simulink model "quadrotorsmodel2"  (R2025b)
settings: Solver=FixedStepAuto  StartTime=0.0  StopTime=SimulationTime  FixedStep=timestep  RelTol=1e-3
values from neighbouring files (symbols this model uses):
  alt_init = 0    [data_hard.mat]
  fense_lats = [14.294404 14.301206]    [data_hard.mat]
  fense_lons = [101.16723 101.176794]    [data_hard.mat]
  g = 9.81    [Copy_of_TESA_Workspace2.m]    (also in TESA_Workspace2.m)
  I = eye(3,3)    [Copy_of_TESA_Workspace2.m]    (also in TESA_Workspace2.m)
  K = [ 1   1   1   1 ... (first row only)    [Copy_of_TESA_Workspace2.m]    (also in TESA_Workspace2.m)
  lat_init = 14.303    [data_hard.mat]
  long_init = 101.155    [data_hard.mat]
  m = 4.34    [Copy_of_TESA_Workspace2.m]    (also in TESA_Workspace2.m)
undefined symbols (not defined in the file or in its folder): dspblkCoreblockFVToolHelper, fractalcoef, gcbh, Kp, Kr, Kv, Kw
libraries: sensorgpslib x1, mspsensorlib x1
settings Model: Creator=worap  LastModifiedBy=Gigabyte
settings DataIOCC: ExternalInput=inputStructure  LoadExternalInput=on

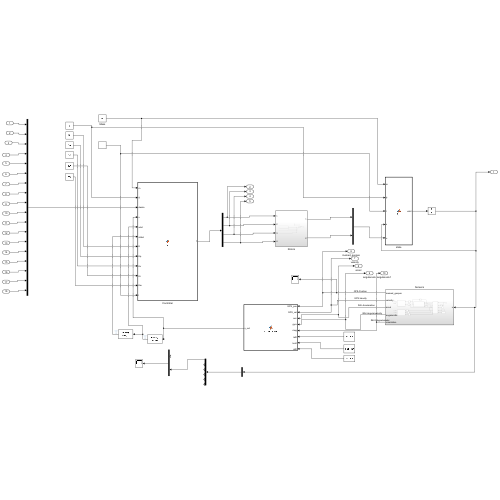
[thumbnail: Simulink's stored preview of the top-level diagram]
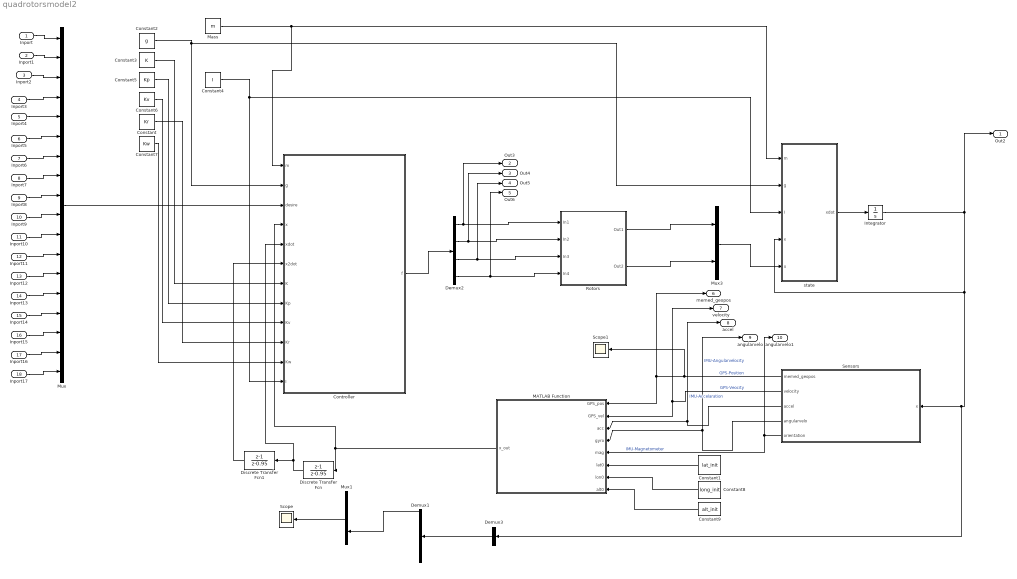
== system quadrotorsmodel2 ==
  Inport : Inport
  Inport1 : Inport  Port=2
  Inport2 : Inport  Port=3
  Inport3 : Inport  Port=4
  Inport4 : Inport  Port=5
  Inport5 : Inport  Port=6
  Inport6 : Inport  Port=7
  Inport7 : Inport  Port=8
  Inport8 : Inport  Port=9
  Inport9 : Inport  Port=10
  Inport10 : Inport  Port=11
  Inport11 : Inport  Port=12
  Inport12 : Inport  Port=13
  Inport13 : Inport  Port=14
  Inport14 : Inport  Port=15
  Inport15 : Inport  Port=16
  Inport16 : Inport  Port=17
  Inport17 : Inport  Port=18
  Constant : Constant  Value=Kr
  Constant1 : Constant  Value=lat_init
  Constant2 : Constant  Value=g
  Constant3 : Constant  Value=K
  Constant4 : Constant  Value=I
  Constant5 : Constant  Value=Kp
  Constant6 : Constant  Value=Kv
  Constant7 : Constant  Value=Kw
  Constant8 : Constant  Value=long_init
  Constant9 : Constant  Value=alt_init
  Controller : MATLAB Function  TreatAsAtomicUnit=on
  Demux1 : Demux  Outputs=6
  Demux2 : Demux
  Demux3 : Demux  Outputs=1
  Discrete Transfer Fcn : DiscreteTransferFcn  LoadFcn=dspblkCoreblockFVToolHelper(gcbh,'load');  Numerator="[1  -1]"  Denominator="[1  -0.95]"  InitialStates=0.01
      settings: CopyFcn=dspblkCoreblockFVToolHelper(gcbh,'copy');  DeleteFcn=dspblkCoreblockFVToolHelper(gcbh,'close');  ModelCloseFcn=dspblkCoreblockFVToolHelper(gcbh,'close');  PreSaveFcn=dspblkCoreblockFVToolHelper(gcbh,'presave');  PostSaveFcn=dspblkCoreblockFVToolHelper(gcbh,'postsave');  CloseFcn=dspblkCoreblockFVToolHelper(gcbh,'close');
  Discrete Transfer Fcn1 : DiscreteTransferFcn  LoadFcn=dspblkCoreblockFVToolHelper(gcbh,'load');  Numerator="[1  -1]"  Denominator="[1  -0.95]"  InitialStates=0.01
      settings: CopyFcn=dspblkCoreblockFVToolHelper(gcbh,'copy');  DeleteFcn=dspblkCoreblockFVToolHelper(gcbh,'close');  ModelCloseFcn=dspblkCoreblockFVToolHelper(gcbh,'close');  PreSaveFcn=dspblkCoreblockFVToolHelper(gcbh,'presave');  PostSaveFcn=dspblkCoreblockFVToolHelper(gcbh,'postsave');  CloseFcn=dspblkCoreblockFVToolHelper(gcbh,'close');
  Integrator : Integrator  InitialCondition=[0;0;0;0;0;0;1;0;0;0;1;0;0;0;1;0;0;0]
  MATLAB Function : MATLAB Function  TreatAsAtomicUnit=on
  Mass : Constant  Value=m
  Mux : Mux  Inputs=18
  Mux1 : Mux  Inputs=2
  Mux3 : Mux  Inputs=2
  Rotors : Subsystem
  Scope : Scope
      settings: ActiveDisplayYMinimum=-1789.9407  ActiveDisplayYMaximum=2269.5419
  Scope1 : Scope
      settings: ActiveDisplayYMinimum=-1789.9407  ActiveDisplayYMaximum=2269.5419
  Sensors : Subsystem
  state : MATLAB Function  TreatAsAtomicUnit=on
  Out2 : Outport
  Out3 : Outport  Port=2
  Out4 : Outport  Port=3
  Out5 : Outport  Port=4
  Out6 : Outport  Port=5
  memed_geopos : Outport  Port=6
  velocity : Outport  Port=7
  accel : Outport  Port=8
  angularvelo : Outport  Port=9
  angularvelo1 : Outport  Port=10
  wires:
  Mass/1 -> state/1(m), Controller/1(m)
  Demux2/2 -> Out4/1, Rotors/2(In2)
  Rotors/1(Out1) -> Mux3/1
  Rotors/2(Out2) -> Mux3/2
  Demux2/3 -> Out5/1, Rotors/3(In3)
  Demux2/4 -> Out6/1, Rotors/4(In4)
  Constant4/1 -> state/3(I), Controller/12(I)
  Controller/1(f) -> Demux2/1
  Demux2/1 -> Out3/1, Rotors/1(In1)
  Constant2/1 -> state/2(g), Controller/2(g)
  Constant3/1 -> Controller/7(K)
  Constant5/1 -> Controller/8(Kp)
  Constant6/1 -> Controller/9(Kv)
  Constant7/1 -> Controller/11(Kw)
  Constant/1 -> Controller/10(Kr)
  Mux3/1 -> state/5(u)
  state/1(xdot) -> Integrator/1
  Mux/1 -> Controller/3(desire)
  Inport17/1 -> Mux/18
  Inport16/1 -> Mux/17
  Inport15/1 -> Mux/16
  Inport14/1 -> Mux/15
  Inport13/1 -> Mux/14
  Inport12/1 -> Mux/13
  Inport11/1 -> Mux/12
  Inport10/1 -> Mux/11
  Inport9/1 -> Mux/10
  Inport8/1 -> Mux/9
  Inport7/1 -> Mux/8
  Inport6/1 -> Mux/7
  Inport5/1 -> Mux/6
  Inport4/1 -> Mux/5
  Inport3/1 -> Mux/4
  Inport2/1 -> Mux/3
  Inport1/1 -> Mux/2
  Inport/1 -> Mux/1
  Sensors/1(memed_geopos) -> Scope1/1, MATLAB Function/1(GPS_pos), memed_geopos/1  "GPS-Position"
  Sensors/2(velocity) -> MATLAB Function/2(GPS_vel), velocity/1  "GPS-Veocity"
  Sensors/3(accel) -> MATLAB Function/3(acc), accel/1  "IMU-Accelaration"
  Sensors/4(angularvelo) -> angularvelo/1, MATLAB Function/4(gyro)  "IMU-Angularvelocity"
  Sensors/5(orientation) -> MATLAB Function/5(mag), angularvelo1/1  "IMU-Magnetometer"
  Discrete Transfer Fcn1/1 -> Controller/6(x2dot)
  Integrator/1 -> Demux3/1, Sensors/1(x), state/4(x), Out2/1
  Mux1/1 -> Scope/1
  MATLAB Function/1(x_out) -> Controller/4(x), Discrete Transfer Fcn/1
  Constant1/1 -> MATLAB Function/6(lat0)
  Constant8/1 -> MATLAB Function/7(lon0)
  Constant9/1 -> MATLAB Function/8(alt0)
  Demux1/1 -> Mux1/2
  Demux3/1 -> Demux1/1
  Discrete Transfer Fcn/1 -> Controller/5(xdot), Discrete Transfer Fcn1/1

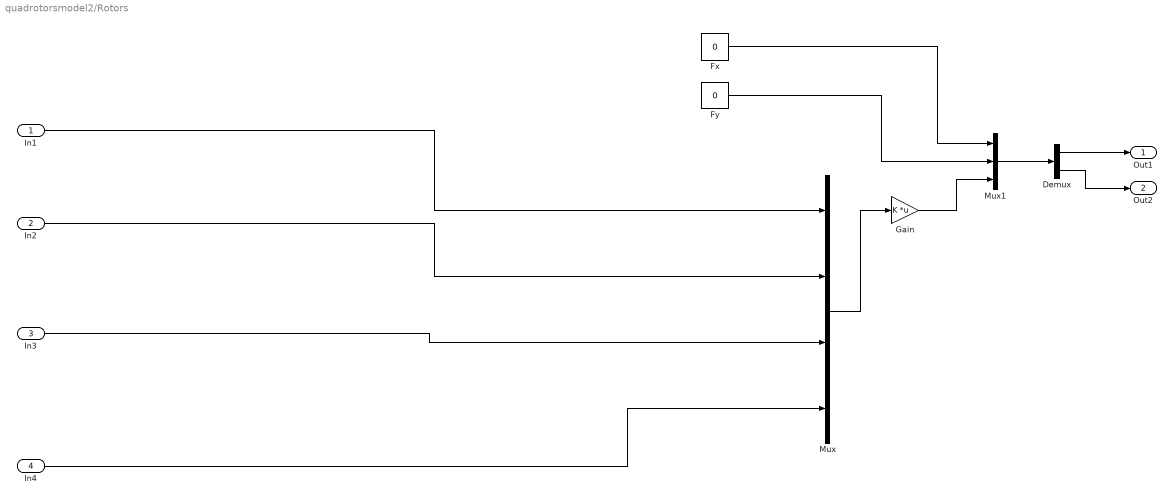
== system quadrotorsmodel2/Rotors ==
  In1 : Inport
  In2 : Inport  Port=2
  In3 : Inport  Port=3
  In4 : Inport  Port=4
  Demux : Demux  Outputs=2
  Fx : Constant  Value=0
  Fy : Constant  Value=0
  Gain : Gain  Gain=K  Multiplication=Matrix(K*u) (u vector)
  Mux : Mux
  Mux1 : Mux  Inputs=3
  Out1 : Outport
  Out2 : Outport  Port=2
  wires:
  Fx/1 -> Mux1/1
  Mux1/1 -> Demux/1
  Fy/1 -> Mux1/2
  Mux/1 -> Gain/1
  Gain/1 -> Mux1/3
  Demux/2 -> Out2/1
  Demux/1 -> Out1/1
  In1/1 -> Mux/1
  In2/1 -> Mux/2
  In3/1 -> Mux/3
  In4/1 -> Mux/4

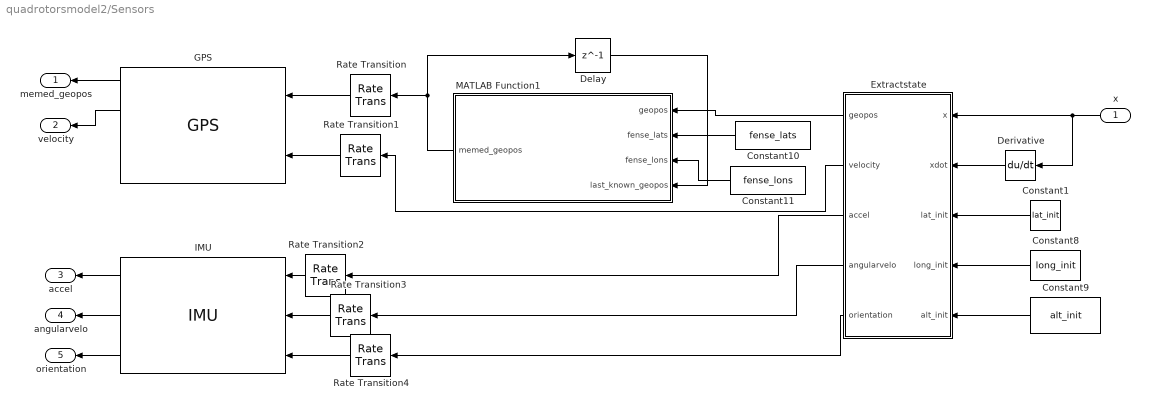
== system quadrotorsmodel2/Sensors ==
  x : Inport
  Constant1 : Constant  Value=lat_init
  Constant10 : Constant  Value=fense_lats
  Constant11 : Constant  Value=fense_lons
  Constant8 : Constant  Value=long_init
  Constant9 : Constant  Value=alt_init
  Delay : Delay  DelayLength=1  InitialCondition=0
  Derivative : Derivative
  Extractstate : MATLAB Function  TreatAsAtomicUnit=on
  GPS : sensorgpslib/GPS  DispRefFrame=NED  PositionInputFormat=Geodetic  ReferenceLocation=[ 0, 0, 0 ]  HorizontalPositionAccuracy=1.6  VerticalPositionAccuracy=3  VelocityAccuracy=0.1  DecayFactor=0.999  SeedDouble=67  SimulateUsing=Interpreted execution
      settings: LibrarySourceBlock=mspsensorlib/GPS
  IMU : mspsensorlib/IMU  DispRefFrame=NED  TemperaturePort=off  Temperature=25  MagneticFieldPort=off  MagneticFieldNED=[ 27.5550, -2.4169, -16.0849 ]  MagneticFieldENU=[ -2.4169, 27.5550, 16.0849 ]  SeedDouble=67  SimulateUsing=Interpreted execution  AccelParamsMeasurementRange=Inf  AccelParamsResolution=0  AccelParamsConstantBias=[ 0, 0, 0 ]  AccelParamsAxesMisalignment=[ 100, 0, 0; 0, 100, 0; 0, 0, 100 ]  AccelParamsNoiseDensity=[ 0.003924 0.003924 0.003924 ]  AccelParamsBiasInstability=[ 0, 0, 0 ]  AccelParamsBiasInstabilityNumerator=fractalcoef().Numerator  AccelParamsBiasInstabilityDenominator=fractalcoef().Denominator  AccelParamsRandomWalk=[ 0, 0, 0 ]  AccelParamsNoiseType=double-sided  AccelParamsTemperatureBias=[ 0, 0, 0 ]  AccelParamsTemperatureScaleFactor=[ 0, 0, 0 ]  GyroParamsMeasurementRange=Inf  GyroParamsResolution=0  GyroParamsConstantBias=[ 0, 0, 0 ]  GyroParamsAxesMisalignment=[ 100, 0, 0; 0, 100, 0; 0, 0, 100 ]  GyroParamsAccelerationBias=[ 0, 0, 0 ]  GyroParamsNoiseDensity=[ 0.0125, 0.0125, 0.0125 ]  GyroParamsBiasInstability=[ 0, 0, 0 ]  GyroParamsBiasInstabilityNumerator=fractalcoef().Numerator  GyroParamsBiasInstabilityDenominator=fractalcoef().Denominator  GyroParamsRandomWalk=[ 0, 0, 0 ]  GyroParamsNoiseType=double-sided  GyroParamsTemperatureBias=[ 0, 0, 0 ]  GyroParamsTemperatureScaleFactor=[ 0, 0, 0 ]  MagParamsMeasurementRange=Inf  MagParamsResolution=0  MagParamsConstantBias=[ 0, 0, 0 ]  MagParamsAxesMisalignment=[ 100, 0, 0; 0, 100, 0; 0, 0, 100 ]  MagParamsNoiseDensity=[0.6 0.6 0.9]/sqrt(100)  MagParamsBiasInstability=[ 0, 0, 0 ]  MagParamsBiasInstabilityNumerator=fractalcoef().Numerator  MagParamsBiasInstabilityDenominator=fractalcoef().Denominator  MagParamsRandomWalk=[ 0, 0, 0 ]  MagParamsNoiseType=double-sided  MagParamsTemperatureBias=[ 0, 0, 0 ]  MagParamsTemperatureScaleFactor=[ 0, 0, 0 ]
  MATLAB Function1 : MATLAB Function  TreatAsAtomicUnit=on
  Rate Transition{,1..4} (5 alike) : RateTransition
  memed_geopos : Outport
  velocity : Outport  Port=2
  accel : Outport  Port=3
  angularvelo : Outport  Port=4
  orientation : Outport  Port=5
  wires:
  Constant11/1 -> MATLAB Function1/3(fense_lons)
  Constant8/1 -> Extractstate/4(long_init)
  Constant1/1 -> Extractstate/3(lat_init)
  Constant10/1 -> MATLAB Function1/2(fense_lats)
  Delay/1 -> MATLAB Function1/4(last_known_geopos)
  Derivative/1 -> Extractstate/2(xdot)
  Constant9/1 -> Extractstate/5(alt_init)
  MATLAB Function1/1(memed_geopos) -> Rate Transition/1, Delay/1
  x/1 -> Derivative/1, Extractstate/1(x)
  IMU/1 -> accel/1
  IMU/2 -> angularvelo/1
  IMU/3 -> orientation/1
  Extractstate/3(accel) -> Rate Transition2/1
  Extractstate/4(angularvelo) -> Rate Transition3/1
  Extractstate/5(orientation) -> Rate Transition4/1
  Extractstate/2(velocity) -> Rate Transition1/1
  GPS/1 -> memed_geopos/1
  GPS/2 -> velocity/1
  Rate Transition/1 -> GPS/1
  Rate Transition1/1 -> GPS/2
  Rate Transition2/1 -> IMU/1
  Rate Transition3/1 -> IMU/2
  Rate Transition4/1 -> IMU/3
  Extractstate/1(geopos) -> MATLAB Function1/1(geopos)

== matlab function quadrotorsmodel2/state ==
  data: m input; g input; I input; x input; u input; xdot output
function xdot = fcn(m,g,I,x,u)

% extract the x-vextor
p = x(1:3,1);
v = x(4:6,1);
R = reshape(x(7:15,1),3,3);
omega = x(16:18,1);

%control signal
f = u(3,1);
M = u(4:6,1);

e3 = [0;0;1];


xdot = zeros(size(x));

xdot(1:3,1) = v;
xdot(4:6,1) = g*e3 - 1/m*f*R*e3;

Rdot = R*hatmap(omega);
xdot(7:15,1) = Rdot(:);

xdot(16:18,1) = I\(M - cross(omega,I*omega));




end

== matlab function quadrotorsmodel2/Controller ==
  data: m input; g input; f output; desire input; x input; xdot input; x2dot input; K input; Kp input; Kv input; Kr input; Kw input; I input
function f  = fcn(m,g,desire,x,xdot,x2dot,K,Kp,Kv,Kr,Kw,I)
%==========================================================================
% Quadrotor Controller (Unclamped version)
% Coordinate: NED (+Z down)
%==========================================================================
% Inputs:
%   m,g,K,Kp,Kv,Kr,Kw,I : physical and control parameters
%   desire : desired trajectory [x y z dx dy dz ddx ddy ddz psi dpsi ddpsi]
%   x, xdot : current state and velocity
% Output:
%   f : [f1; f2; f3; f4] motor thrusts (unbounded)
%   Phee_value : desired yaw (for plotting)
%==========================================================================

%% === Desired trajectory ===
xt = desire(1); yt = desire(2); zt = desire(3);
dxt = desire(4); dyt = desire(5); dzt = desire(6);
ddxt = desire(7); ddyt = desire(8); ddzt = desire(9);
psit  = desire(16); dpsit = desire(17); ddpsit = desire(18);

rt   = [xt; yt; zt];
drt  = [dxt; dyt; dzt];
d2rt = [ddxt; ddyt; ddzt];

%% === Current state ===
r   = x(1:3);
dr  = xdot(1:3);
R   = reshape(x(7:15),3,3);
omega = x(16:18,1);

% --- Normalize rotation matrix
[U,~,V] = svd(R);
R = U*V';

%% === Outer-loop Position Control ===
ep = r - rt;
ev = dr - drt;

% Desired acceleration (Feedforward + PD)
a_des = d2rt - Kp * ep - Kv * ev;

% Safety check (only for NaN/Inf)
if (any(isnan(a_des(:))) || any(isinf(a_des(:))))
    a_des = zeros(3,1);
end

%% === Desired force (NED frame) ===
g_vec = [0; 0; g];
F_des = m * (g_vec - a_des);

if any(isnan(F_des)) || any(isinf(F_des)) || norm(F_des) < 1e-6
    F_des = [0; 0; m*g];
end

%% === Compute total thrust ===
f_total = dot(F_des, R(:,3));  % no clamping

%% === Desired attitude ===
zb_des = F_des / (norm(F_des) + 1e-6);
xc_des = [cos(psit); sin(psit); 0];

% Avoid singularity when zb_des || xc_des
if norm(cross(zb_des, xc_des)) < 1e-6
    xc_des = [ -sin(psit); cos(psit); 0 ];
end

yb_des = cross(zb_des, xc_des);
yb_des = yb_des / (norm(yb_des) + 1e-6);
xb_des = cross(yb_des, zb_des);
R_des = [xb_des, yb_des, zb_des];

%% === Attitude Control ===
omega_des = [0; 0; dpsit];

e_Rm = 0.5 * (R_des' * R - R' * R_des);
e_R = [e_Rm(3,2); e_Rm(1,3); e_Rm(2,1)];
e_omega = omega - R' * R_des * omega_des;

% Full torque control law
tau = -Kr * e_R - Kw * e_omega + cross(omega, I*omega);

%% === Motor Mixing ===
invK = pinv(K);
u_vec = [f_total; tau(1); tau(2); tau(3)];
f = invK * u_vec;  % no clamping

% last safety check
if any(isnan(f(:))) || any(isinf(f(:))) || any(~isfinite(f(:)))
    f = zeros(4,1);
end

%% === Outputs ===
% Phee_value = psit;

end

== matlab function quadrotorsmodel2/Sensors/Extractstate ==
  data: geopos output; velocity output; x input; accel output; xdot input; angularvelo output; orientation output; lat_init input; long_init input; alt_init input
function [geopos, velocity,accel, angularvelo, orientation] = Extractstate(x,xdot,lat_init,long_init,alt_init)

position = x(1:3)';
velocity = x(4:6)';
accel = xdot(4:6)';
R = x(7:15);
orientation = reshape(R,3,3);
angularvelo = x(16:18)';


geopos = ned2lla(position, [lat_init long_init alt_init], "ellipsoid");

end

== matlab function quadrotorsmodel2/Sensors/MATLAB Function1 ==
  data: geopos input; memed_geopos output; fense_lats input; fense_lons input; last_known_geopos input
function memed_geopos  = is_jammed(geopos, fense_lats, fense_lons, last_known_geopos)
    
    memed_geopos = geopos;

    if fense_lats ~= 0
        if (geopos(1) > min(fense_lats)) && (geopos(1) < max(fense_lats)) && (geopos(2) > min(fense_lons)) && (geopos(2) < max(fense_lons))
            memed_geopos = [14.30613815134626, 101.18904132968885, 30];
        end
    end
end

== matlab function quadrotorsmodel2/MATLAB Function ==
  data: GPS_pos input; GPS_vel input; acc input; gyro input; x_out output; mag input; lat0 input; lon0 input; alt0 input
function x_out = sensorFusion(GPS_pos, GPS_vel, acc, gyro, mag, lat0, lon0, alt0)
% =========================================================================
%   Sensor Fusion v3 (Filter-only, no spoof injection)
%   - Accept possibly-false GPS, detect & reject internally
%   - GPS jump rejection + recovery state machine
%   - GPS freeze/spoof detection (false fixed position)
%   - Gyro propagation + acc/mag correction (complementary AHRS)
%   - Complementary fusion for pos/vel
%   Frame: NED (+Z down), R maps body -> NED
%   Output 18x1 matches your controller:
%     1:3 pos, 4:6 vel, 7:15 R(:), 16:18 gyro
% =========================================================================

x_out = zeros(18,1);

persistent pos vel last_good_gps gps_state stable_count initialized
persistent R_est gyro_bias acc_lpf mag_lpf gps_prev gps_freeze_count

if isempty(initialized)
    pos = [0;0;0];
    vel = [0;0;0];

    last_good_gps = [0;0;0];
    gps_prev = [0;0;0];

    gps_state = 0;        % 0=GOOD, 1=REJECTED(jump/bad), 2=RECOVERING, 3=JAMMED(freeze)
    stable_count = 0;
    gps_freeze_count = 0;

    R_est = eye(3);
    gyro_bias = [0;0;0];

    acc_lpf = [0;0;0];
    mag_lpf = [1;0;0];

    initialized = true;
end

%% PARAMETERS ===============================================================
dt = 0.01;      % should match Simulink Ts
g  = 9.81;
Re = 6378137;

% --- GPS jump / recovery thresholds
jump_threshold    = 200;    % meters
recover_threshold = 80;     % meters
recover_cycles    = 3;

% --- Complementary fusion weights
alpha_pos_good = 0.04;
alpha_vel_good = 0.10;
alpha_pos_bad  = 0.003;
alpha_vel_bad  = 0.003;

% --- LPF for IMU
alpha_acc_lpf = 0.25;
alpha_mag_lpf = 0.20;

% --- Attitude complementary gains
k_acc = 0.08;   % roll/pitch correction
k_mag = 0.04;   % yaw correction

% --- Freeze / false-fixed GPS detection thresholds
pos_freeze_thr   = 0.5;    % m, GPS position barely changes
vel_freeze_thr   = 0.3;    % m/s, GPS vel near zero
acc_motion_thr   = 0.4;    % m/s^2, IMU indicates translation
gyro_motion_thr  = 0.035;  % rad/s, IMU indicates rotation (~2 deg/s)
freeze_cycles    = 10;     % consecutive cycles -> JAMMED

%% 0) LPF IMU ==============================================================
acc  = acc(:); gyro = gyro(:); mag = mag(:);

acc_lpf = (1-alpha_acc_lpf)*acc_lpf + alpha_acc_lpf*acc;
mag_lpf = (1-alpha_mag_lpf)*mag_lpf + alpha_mag_lpf*mag;
if norm(mag_lpf) < 1e-6, mag_lpf = [1;0;0]; end

%% 1) Convert raw GPS -> NED ===============================================
GPS_valid = ~(any(isnan(GPS_pos)) || any(isinf(GPS_pos)));

if GPS_valid
    dLat = (GPS_pos(1) - lat0) * pi/180;
    dLon = (GPS_pos(2) - lon0) * pi/180;

    px = dLat * Re;
    py = dLon * Re * cos(lat0*pi/180);
    pz = -(GPS_pos(3) - alt0);

    gps_ned = [px; py; pz];
else
    gps_ned = last_good_gps;
end

%% 2) Detect GPS freeze / false-fixed spoof ===============================
% Condition: GPS position ~ constant AND GPS vel ~ 0 BUT IMU says moving

pos_static = norm(gps_ned - gps_prev) < pos_freeze_thr;

if any(isnan(GPS_vel)) || any(isinf(GPS_vel))
    vel_static = true;  % vel unreliable -> treat as static
else
    vel_static = norm(GPS_vel(:)) < vel_freeze_thr;
end

imu_motion = (norm(acc_lpf) > acc_motion_thr) || (norm(gyro) > gyro_motion_thr);

if pos_static && vel_static && imu_motion
    gps_freeze_count = gps_freeze_count + 1;
else
    gps_freeze_count = 0;
end

freeze_jam_flag = gps_freeze_count >= freeze_cycles;
gps_prev = gps_ned;

%% 3) GPS state machine (jump + jam + recovery) ===========================
dist_jump = norm(gps_ned - last_good_gps);

switch gps_state
    case 0   % GOOD
        if freeze_jam_flag
            gps_state = 3;  % JAMMED
            stable_count = 0;

        elseif (~GPS_valid) || (dist_jump > jump_threshold)
            gps_state = 1;  % REJECTED (jump/bad)
            stable_count = 0;
        end

    case 1   % REJECTED
        if freeze_jam_flag
            gps_state = 3;
            stable_count = 0;

        elseif GPS_valid && dist_jump < recover_threshold
            gps_state = 2;  % RECOVERING
            stable_count = 1;
        end

    case 2   % RECOVERING
        if freeze_jam_flag
            gps_state = 3;
            stable_count = 0;

        elseif ~GPS_valid
            gps_state = 1;
            stable_count = 0;

        elseif dist_jump < recover_threshold
            stable_count = stable_count + 1;
            if stable_count >= recover_cycles
                gps_state = 0;
                last_good_gps = gps_ned;
            end
        else
            gps_state = 1;
            stable_count = 0;
        end

    case 3   % JAMMED (false fixed)
        % Exit jam when GPS starts changing again consistently
        if GPS_valid && (~pos_static)
            gps_state = 2;
            stable_count = 1;
            gps_freeze_count = 0;
        end
end

%% 4) Choose GPS for fusion ================================================
if gps_state == 0
    gps_used = gps_ned;
    last_good_gps = gps_ned;
    alpha_pos = alpha_pos_good;
    alpha_vel = alpha_vel_good;

elseif gps_state == 2
    gps_used = gps_ned;  % soft return
    alpha_pos = alpha_pos_bad;
    alpha_vel = alpha_vel_bad;

else
    % REJECTED or JAMMED -> freeze last_good_gps
    gps_used = last_good_gps;
    alpha_pos = alpha_pos_bad;
    alpha_vel = alpha_vel_bad;
end

%% 5) AHRS: gyro propagation + acc/mag correction ==========================
omega = gyro - gyro_bias;

Omega = [   0     -omega(3)  omega(2);
          omega(3)    0     -omega(1);
         -omega(2) omega(1)    0    ];

R_pred = R_est * expm(Omega*dt);

% Acc correction (gravity alignment)
acc_b = acc_lpf;
if norm(acc_b) > 1e-6
    z_b = acc_b / norm(acc_b);
    z_n = R_pred(:,3);
    e_acc = cross(z_n, R_pred*z_b);
else
    e_acc = [0;0;0];
end

% Mag correction (tilt compensated yaw)
m_n = R_pred * (mag_lpf / norm(mag_lpf));
m_h = [m_n(1); m_n(2); 0];
if norm(m_h) > 1e-6, m_h = m_h / norm(m_h); end
e_mag = cross([1;0;0], m_h);

E = k_acc*skew(e_acc) + k_mag*skew(e_mag);
R_est = (eye(3) + E) * R_pred;

% Orthonormalize
[U,~,V] = svd(R_est);
R_est = U*V';

%% 6) Rotate acc to NED ====================================================
acc_ned = R_est * acc_b - [0;0;g];
if any(~isfinite(acc_ned)), acc_ned = [0;0;0]; end

%% 7) IMU prediction =======================================================
pos_pred = pos + vel*dt + 0.5*acc_ned*dt*dt;
vel_pred = vel + acc_ned*dt;

%% 8) Complementary fusion =================================================
pos = (1-alpha_pos)*pos_pred + alpha_pos * gps_used;

if any(isnan(GPS_vel)) || any(isinf(GPS_vel))
    vel_gps_used = vel_pred;
else
    vel_gps_used = GPS_vel(:);
end
vel = (1-alpha_vel)*vel_pred + alpha_vel * vel_gps_used;

%% 9) Output ===============================================================
x_out(1:3)   = pos;
x_out(4:6)   = vel;
x_out(7:15)  = R_est(:);
x_out(16:18) = gyro(:);

end

function S = skew(v)
S = [    0, -v(3),  v(2);
      v(3),    0, -v(1);
     -v(2), v(1),    0 ];
end
